simulink model "eVTOL_Small_nonandlin_algorithm_validation"  (R2024b)
settings: Solver=ode3  StartTime=0.0  StopTime=220  FixedStep=0.02  RelTol=1e-3
undefined symbols (not defined in the file): a_, b, c, c1_, deg, dttrim0, F, g, g1, h1, l1, m, MIL, PARAR, rad, rho, s, T, u_dim, ut, x_dim, xf, xmset, y_dim, yf, ymset, zf, zmset
libraries: simulink x34, aerolibconvert2 x5, aerolibwind2 x2, shared6dof x1
(part 6 of 7)

== matlab function eVTOL_Small_nonandlin_algorithm_validation/各部件气动力和力矩/8组旋翼模块/旋翼组7/上旋翼7  ==
  data: FMx output; omegaset input; u input; v input; w input; p input; q input; r input; xmset input; ymset input; zmset input; PARAR input; FMy output; FMz output; MMx output; MMy output; MMz output; PSR output; viU output; AEOCTB output
 function [FMx, FMy, FMz, MMx, MMy, MMz, PSR, viU, AEOCTB] = ROTOR7U(omegaset,u,v,w,p,q,r,xmset,ymset,zmset,PARAR) 

 % omegaset(7)为第七组上旋翼
 omega = omegaset(7);
  
 % 需要的无量纲和旋翼参数
 kt = 0.01;
 
 d2r = 0.017453292;
 
 rho = PARAR(1);
 eta = PARAR(2);
 g   = PARAR(3);
 
 nbMR     =  PARAR(4);                   % 桨叶片数(Number of blades)
 RM       =  PARAR(5);                   % 桨叶半径(Rotor radius), m
 cMR      =  PARAR(6);                   % 桨叶弦长(Blade root chord), m
 eMR      =  PARAR(7);                   % 挥舞铰偏置量(Flapping hinge offset), m
 isMR     =  PARAR(8);                   % 旋翼前倾角(Rotor shaft tilt), rad
 MbMR     =  PARAR(9);                   % 单片桨叶关于挥舞铰的质量矩(Mass moment of blade about flapping hinge), kg*m
 IbMR     =  PARAR(10);                  % 单片桨叶关于挥舞铰的惯性矩(Inertia moment of blade about flapping hinge), kg*m^2
 KindMRU  =  PARAR(11);                  % 上旋翼诱导功率修正系数;
 interU   =  PARAR(12);                  % 上旋翼诱导速度修正系数;
 interL   =  PARAR(13);                  % 下旋翼诱导速度修正系数;
 KindMR   =  PARAR(14);                  % 诱导功率修正系数(Induced power factor)
 XKBR     =  PARAR(15);                  % 桨叶挥舞弹簧系数(N-M/RAD)
 theta1MR =  PARAR(16);                  % 桨叶扭转角(Blade twist), rad
 aMR      =  PARAR(17);                  % 桨叶升力线斜率(Blade lift curve slope)
 cdMR     =  PARAR(18);                  % 单片桨叶的型阻系数(Blade profile drag coefficient)
 kBLADE   =  PARAR(19);                  % 叶端损失系数
 sigmaMR  =  PARAR(20);                  % 旋翼实度(Rotor solidity)
 gamaMR   =  PARAR(21);                  % 桨叶洛克数(Blade Lock number)

 xm = xmset(7); % 旋翼桨毂中心位置，第七组旋翼
 ym = ymset(7);
 zm = zmset(7);
 
 theta0 = PARAR(22);
 thetac = PARAR(23);
 thetas = PARAR(24);
 
 % 1.体轴系重心速度 转换到 体轴系桨毂处的速度
 uM  = u + (zm*q - ym*r);
 vM  = v + (xm*r - zm*p);
 wM  = w + (ym*p - xm*q);
 
 % 2.体轴系桨毂处的速度 转换到 桨毂轴系速度（无量纲）  直升机运动速度，不是风的速度
 muxB = ( uM*cos(isMR) + wM*sin(isMR) )/(omega*RM);   % m/s /(omega*RM)
 muyB = ( vM )/(omega*RM);                            % m/s /(omega*RM)
 muzB = (-uM*sin(isMR) + wM*cos(isMR) )/(omega*RM);   % m/s /(omega*RM)
 
 % 3.体轴系桨毂处的角速度 转换到 桨毂轴系角速度（无量纲） 确定旋翼锥度角、后倒角和侧倾角,还有后向力系数与侧向力系数
 wxB  = ( p*cos(isMR) + r*sin(isMR) )/omega;    % rad/s /(omega)
 wyB  = ( q )/omega;
 %wzB  = (-p*sin(isMR) + r*cos(isMR) )/omega;
 
 % 4.初始化：确定UcB(垂直向下)，UtB(平行)
 CTB1 = 1; % CTB牛顿迭代初始值
 
 UcB  = -muzB / ( sqrt(kt*CTB1/2.d0) ); % sqrt(CT/2)*omega*R为悬停时候的诱导速度，UcB为风的速度，方向和桨毂运动速度相反，所以加上负号，搞不清楚可以假设前上飞，此时UcB一定大于0
 UtB  = sqrt(muxB^2 + muyB^2) / ( sqrt(kt*CTB1/2.d0) ); % 照道理也要添加负号，不过后面用的是Ut的平方，所以加不加负号无所谓
 
 % 5.初始化：确定诱导速度比
 if( (2.d0*UcB+3.d0)^2 + UtB*UtB >1.d0 )         % 滑流理论适用，Newton－Raphson方法迭代求解，Johson提出的涡环状态下经验估计
     viB = N_R ( UcB, UtB );                     % N_R为迭代函数
 else
     viB = UcB * ( 0.373d0*UcB*UcB + 0.598d0*UtB*UtB - 1.991d0 );
 end
 viB = viB*interU;                               % 上旋翼诱导速度修正
 
 % 6.初始化：确定fG、lammda1(无量纲)、诱导速度和AEOCTB（代数方程右端项）
 %lammda = ( UcB+viB ) * sqrt(kt*CTB1/2.d0);                % 入流速度 /(omega*RM)
 %zh      = hB*k3*RM + HR - drotor;
 mu     = sqrt(muxB^2+muyB^2);                             % /(omega*RM)
 fG     = 1.0d0; %- sigmaMR*aMR*lammda/(4.d0*kt*CTB1) * (RM/(4.d0*z))**2/( 1.d0 + (mu/lammda)**2 )
 lammda1= muzB - viB * sqrt(kt*CTB1/2.d0) * fG * KindMRU;  % 向下为正，若直升机向上飞 则muzB为负
  
 AEOCTB1  = kt*CTB1 - 0.5d0*kBLADE*aMR*sigmaMR*((1.d0/3.d0 + 0.5d0*mu^2)*theta0...
     + 0.25d0*(1.0d0 + mu^2)*theta1MR + 0.5d0*lammda1...
     - 0.5d0*(muyB*thetac + muxB*thetas) + 0.25d0*(muxB*wxB + muyB*wyB));  %  (与beta0, betac, betas无关，只与theta0, thetac, thetas有关)
 
 % 7.初始化：CTB2 = CTB1 + deltaCTB
 CTB2 = CTB1 + 1e-4;
 
 % 8.进入牛顿迭代：计算配平时候的CTB和vi
 for k = 1:10
     % 计算CTB2下的vi  
     UcB  = -muzB / ( sqrt(kt*CTB2/2.d0) );
     UtB  = sqrt(muxB^2 + muyB^2) / ( sqrt(kt*CTB2/2.d0) );
     if( (2.d0*UcB+3.d0)^2 + UtB*UtB >1.d0 )         
         viB = N_R ( UcB, UtB );                     
     else
         viB = UcB * ( 0.373d0*UcB*UcB + 0.598d0*UtB*UtB - 1.991d0 );
     end
     viB = viB*interU;
     
     % 计算CTB2下的fG、lammda1(无量纲)、诱导速度和AEOCTB（代数方程右端项）
     %lammda = ( UcB+viB ) * sqrt(kt*CTB2/2.d0);            % 入流速度 /(omega*RM)
     %zh      = hB*k3*RM + HR - drotor;
     fG     = 1.d0 ;%- sigmaMR*aMR*lammda/(4.d0*kt*CTB1) * (RM/(4.d0*z))**2/( 1.d0 + (mu/lammda)**2 )
     lammda1= muzB - viB * sqrt(kt*CTB2/2.d0) * fG * KindMRU;  % 向下为正，若直升机向上飞 则muzB为负
     
     AEOCTB2  = kt*CTB2 - 0.5d0*kBLADE*aMR*sigmaMR*((1.d0/3.d0 + 0.5d0*mu^2)*theta0...
         + 0.25d0*(1.0d0 + mu^2)*theta1MR + 0.5d0*lammda1...
         - 0.5d0*(muyB*thetac + muxB*thetas) + 0.25d0*(muxB*wxB + muyB*wyB));  %  (与beta0, betac, betas无关，只与theta0, thetac, thetas有关)
     
     dAEOCTB  =   (AEOCTB2 - AEOCTB1)/(CTB2-CTB1);
     
     AEOCTB1 = AEOCTB2;
     CTB1 = CTB2;
     CTBN = CTB2 - AEOCTB2/dAEOCTB;
     err = abs(CTBN-CTB2);
     relerr = 2*err/(abs(CTBN)+1e-4);
     CTB2 = CTBN;
     
%      % 新CTB2下的vi与AEOCTB（即y）
%      UcB  = -muzB / ( sqrt(kt*CTB2/2.d0) ); % sqrt(CT/2)*omega*R为悬停时候的诱导速度，UcB为风的速度，方向和桨毂运动速度相反，所以加上负号，搞不清楚可以假设前上飞，此时UcB一定大于0
%      UtB  = sqrt(muxB^2 + muyB^2) / ( sqrt(kt*CTB2/2.d0) ); % 照道理也要添加负号，不过后面用的是Ut的平方，所以加不加负号无所谓
%      if( (2.d0*UcB+3.d0)^2 + UtB*UtB >1.d0 )          % 滑流理论适用，Newton－Raphson方法迭代求解，Johson提出的涡环状态下经验估计
%          viB = N_R ( UcB, UtB );                      % N_R为迭代函数
%      else
%          viB = UcB * ( 0.373d0*UcB*UcB + 0.598d0*UtB*UtB - 1.991d0 );
%      end
%      viB = viB*interU;                               % 上旋翼诱导速度修正
%      %lammda = ( UcB+viB ) * sqrt(kt*CTB2/2.d0);     % 入流速度 /(omega*RM)
%      %zh      = hB*k3*RM + HR - drotor;
%      fG     = 1.d0 ;%- sigmaMR*aMR*lammda/(4.d0*kt*CTB1) * (RM/(4.d0*z))**2/( 1.d0 + (mu/lammda)**2 )
%      lammda1= muzB - viB * sqrt(kt*CTB2/2.d0) * fG * KindMR;                      % 向下为正，若直升机向上飞 则muzB为负
%      y = kt*CTB2 - 0.5d0*kBLADE*aMR*sigmaMR*((1.d0/3.d0 + 0.5d0*mu^2)*theta0...
%          + 0.25d0*(1.0d0 + mu^2)*theta1MR + 0.5d0*lammda1...
%          - 0.5d0*(muyB*thetac + muxB*thetas) + 0.25d0*(muxB*wxB + muyB*wyB));
     %if (err<1e-5)||(relerr<1e-5)||(abs(y)<1e-6)
     if (err<1e-4)||(relerr<1e-4)
         break;
     end
 end
 
 CTB = CTB2;
 vim = viB * sqrt(kt*CTB/2.d0) * fG * KindMRU;
 vim = vim*interL;                                 
 viU = vim*omega*RM;                                % 上旋翼诱导速度在下旋翼的发展
 
 AEOCTB = AEOCTB2;
 
 % 9.确定旋翼锥度角、后倒角和侧倾角(用于确定旋翼的后向力和侧向力) 
 Ca1     = 1.d0 - 0.5d0 * mu^2;
 Cb1     = 1.d0 + 0.5d0 * mu^2;
 
 beta0   = 0.5d0*kBLADE*gamaMR * ( 0.25d0*(1+mu^2)*theta0 + (0.2d0+ 1.d0/6.d0 *mu^2)*theta1MR ...
            - 1.d0/3.d0 *muyB*thetac - 1.d0/3.d0 *muxB*thetas + 1.d0/3.d0*lammda1 ...
            + 1.d0/6.d0 *muxB*wxB + 1.d0/6.d0 *muyB*wyB ) - g*MbMR/(IbMR * (omega)^2);
 
 betac   = (8.d0/3.d0 *theta0 + 2.d0*theta1MR + 2.d0*lammda1)*muxB/Ca1 ...
            - 2.d0*muxB*muyB/Ca1 *thetac - (Ca1+2.d0*muxB*muxB)/Ca1 *thetas ...
            + 4.0/(3.d0*Cb1) *muyB*beta0 ...
            + (Cb1 - muyB^2 + 16.d0/(gamaMR*kBLADE)*muxB*muyB) *wxB/(Ca1*Cb1) ...
            + (muxB*muyB - 16.d0/(gamaMR*kBLADE)*(Cb1 - muyB^2)) *wyB/(Ca1*Cb1);
 
 betas   = -(8.d0/3.d0 *theta0 + 2.d0*theta1MR + 2.d0*lammda1)*muyB/Ca1 ...
             + 2.d0*muxB*muyB/Ca1 *thetas + (Ca1+2.d0*muyB*muyB)/Ca1 *thetac ...
             + 4.0/(3.d0*Cb1) *muxB*beta0 ...
            - (Ca1 + muyB^2 - 16.d0/(gamaMR*kBLADE)*muxB*muyB) *wyB/(Ca1*Cb1) ...
            - (muxB*muyB + 16.d0/(gamaMR*kBLADE)*(Ca1 + muyB^2)) *wxB/(Ca1*Cb1);
 
 % 10.确定后向力系数、侧向力系数、需用功率
 CT = CTB*kt;
 
 CH      = 0.25d0*cdMR*sigmaMR*muxB...   % (与beta0, betac, betas, theta0, thetac, thetas均有关)
            + 0.5d0*kBLADE*aMR*sigmaMR*( ...
            (-0.75d0*muyB *beta0 + (1.0/3.d0 + 0.5d0*muyB^2) *betac + 0.5d0*muxB*muyB *betas -0.5d0*muxB*lammda1 -1.d0/6.d0*wxB) *theta0 ...
            + 0.25d0*(-2.d0*muyB *beta0 + (1.d0+muyB^2) *betac + muxB*muyB *betas -muxB*lammda1 - 0.5d0*wxB) *theta1MR ...
            + 0.5d0*((1.d0/3.d0 + muyB^2)*beta0 - muyB*betac + 0.125d0*(muyB*wxB+muxB*wyB)) *thetac ...
            + 0.25d0*(2.d0*muxB*muyB*beta0 - muxB*betac - muyB*betas + lammda1 + 0.75d0*muxB*wxB + 0.25d0*muyB*wyB) *thetas ...
            - muxB*muyB*beta0*betac - (1.d0/6.d0-muyB*muyB)*beta0*betas - 0.25d0*muyB*betac*betas + 0.25d0*muxB*(beta0^2+betac^2) ...
            + 0.75d0*(betac-2.d0*muyB*beta0)*lammda1 ...
            - 0.5d0*(lammda1+0.125d0*muxB*betac-0.875d0*muyB*betas) *wxB - 0.5d0*(1.d0/3.d0*beta0-0.625d0*muyB*betac+0.125d0*muxB*betas) *wyB );
 
 CS      = -0.25d0*cdMR*sigmaMR*muyB ... % (与beta0, betac, betas, theta0, thetac, thetas均有关)
            + 0.5d0*kBLADE*aMR*sigmaMR*( ...
            (-0.75d0*muxB *beta0 + (1.0/3.d0 + 0.5d0*muxB^2) *betas + 0.5d0*muxB*muyB *betac +0.5d0*muyB*lammda1 +1.d0/6.d0*wyB) *theta0 ...
            + 0.25d0*(-2.d0*muxB *beta0 + (1.d0+muxB^2) *betas + muxB*muyB *betac +muyB*lammda1 + 0.5d0*wyB) *theta1MR ...
            + 0.25d0*(2.d0*muxB*muyB *beta0 - muyB *betas - muxB *betac - lammda1 - 0.25d0*muxB*wxB - 0.75d0*muyB*wyB) *thetac ...
            + 0.5d0*((1.0/3.0 + muxB^2) *beta0 - muxB*betas -0.125d0*(muyB*wxB+muxB*wyB)) *thetas ...
            + muxB*muyB*beta0*betas + (1.d0/6.d0-muxB*muxB)*beta0*betac + 0.25d0*muxB*betac*betas - 0.25d0*muyB*(beta0^2+betas^2) ...
            + 0.75d0*(betas-2.d0*muxB*beta0)*lammda1 ...
            + 0.5d0*(lammda1-0.125d0*muyB*betas+0.875d0*muxB*betac) *wyB - 0.5d0*(1.d0/3.d0*beta0-0.625d0*muxB*betas+0.125d0*muyB*betac) *wxB );
 
 CHB      =  CH / kt;
 CSB      =  CS / kt;
 
 CpmB = (-CTB*muzB - CHB*muxB + CSB*muyB)/sqrt(kt) + KindMRU*fG*CTB*sqrt(CTB/2.d0)*viB/interU ...
         + 0.125d0*sigmaMR*cdMR/kt/sqrt(kt)*(1.d0 + 4.7d0*mu^2);

 Cpm = CpmB*(kt*sqrt(kt));
      
 PSR = 1/eta*rho*(pi*RM^2)*(omega*RM)^3*Cpm;
 
 MMk = PSR/omega;
 
 TLHK = nbMR/2.d0 * (XKBR)*betas;
 TMHK = nbMR/2.d0 * (XKBR)*betac;
 
 % 11.确定体轴系下的力和力矩
 FMx =  rho*(pi*RM^2)*(omega*RM)^2 * ( CT*sin(isMR) - CH*cos(isMR) );
 
 FMy =  rho*(pi*RM^2)*(omega*RM)^2 * CS;
 
 FMz = -rho*(pi*RM^2)*(omega*RM)^2 * ( CT*cos(isMR) + CH*sin(isMR) );
 
 MMx = 0.5*nbMR * MbMR * omega^2 * eMR * betas*cos(isMR) - MMk*sin(isMR)  + ( ym*FMz - zm*FMy ) + TLHK*cos(isMR);
 
 MMy = 0.5*nbMR * MbMR * omega^2 * eMR * betac + ( zm*FMx - xm*FMz ) + TMHK;
 
 MMz = 0.5*nbMR * MbMR * omega^2 * eMR * betas*sin(isMR) + MMk*cos(isMR)  + ( xm*FMy - ym*FMx ) + TLHK*sin(isMR);

 
 % 求诱导速度用到的函数
     function p0 = N_R(x_1B,x_2B)
         p0   = 1;
         delta= 0.0001;
         epsilon = 0.0001;
         max1 = 10;
         for k = 1:max1
             p1     = p0-( p0^4+2*x_1B*p0^3+(x_1B^2+x_2B^2)*p0^2-1 )/( 4*p0^3+6*x_1B*p0^2+2*(x_1B^2+x_2B^2)*p0 );
             err    = abs(p1-p0);
             relerr = 2*err/(abs(p1)+delta);
             p0     = p1;
             y      = p0^4+2*x_1B*p0^3+(x_1B^2+x_2B^2)*p0^2-1;
             if (err<delta)||(relerr<delta)||(abs(y)<epsilon)
                 break;
             end
         end

== matlab function eVTOL_Small_nonandlin_algorithm_validation/Voltage_drop ==
  data: Vcoff output; Vcurrent input; dttrim output
function  [Vcoff,dttrim] = voltage_drop(Vcurrent)

Vcurrent1 = Vcurrent + 4;

% 本代码用于压降拟合；
% 根据二代机压降的数据整理可知，相同油门下，转速随电压基本呈现线性变化（详见一二代机压降关系表）；
% 根据零代机的实际试飞情况，满电状态（61V），悬停所需motormax=1.005；低电状态（52V），悬停所需motormax接近1.28（92%油门）；
% 满电状态下的motor与上下旋翼转速之间的关系已经通过旋翼台测得；
% 低电状态下的dt已知，根据线性变化假设，此时悬停对应的转速可以通过满电时候的转速乘以一个系数Vcoff获得（让motormax=1.28时悬停）；
% 最终可以获得低电状态下motor与上下旋翼转速之间的关系，利用不同电压下转速的线性插值，即可反推悬停时候的dt，即不同电压下的dt配平值；

dttrim = 0.0010778*Vcurrent1^2 - 0.14794*Vcurrent1 + 5.888;

Vcoff = 1; %0.011343*Vcurrent1 + 0.30803;

== matlab function eVTOL_Small_nonandlin_algorithm_validation/各部件气动力和力矩/8组旋翼模块/旋翼组7/下旋翼7 ==
  data: FMx output; omegaset input; u input; v input; w input; p input; q input; r input; xmset input; ymset input; zmset input; FMy output; FMz output; MMx output; MMy output; MMz output; PSR output; viL output; AEOCTB output; PARAR input; viU input
 function [FMx, FMy, FMz, MMx, MMy, MMz, PSR, viL, AEOCTB] = ROTOR7L(omegaset,u,v,w,p,q,r,xmset,ymset,zmset,PARAR,viU) 

 % omegaset(15)为第七组下旋翼
 omega = omegaset(15);
  
 % 需要的无量纲和旋翼参数
 kt = 0.01;
 
 d2r = 0.017453292;
 
 rho = PARAR(1);
 eta = PARAR(2);
 g   = PARAR(3);
 
 nbMR     =  PARAR(4);                   % 桨叶片数(Number of blades)
 RM       =  PARAR(5);                   % 桨叶半径(Rotor radius), m
 cMR      =  PARAR(6);                   % 桨叶弦长(Blade root chord), m
 eMR      =  PARAR(7);                   % 挥舞铰偏置量(Flapping hinge offset), m
 isMR     =  PARAR(8);                   % 旋翼前倾角(Rotor shaft tilt), rad
 MbMR     =  PARAR(9);                   % 单片桨叶关于挥舞铰的质量矩(Mass moment of blade about flapping hinge), kg*m
 IbMR     =  PARAR(10);                  % 单片桨叶关于挥舞铰的惯性矩(Inertia moment of blade about flapping hinge), kg*m^2
 KindMR   =  PARAR(14);                  % 诱导功率修正系数(Induced power factor)
 XKBR     =  PARAR(15);                  % 桨叶挥舞弹簧系数(N-M/RAD)
 theta1MR =  PARAR(16);                  % 桨叶扭转角(Blade twist), rad
 aMR      =  PARAR(17);                  % 桨叶升力线斜率(Blade lift curve slope)
 cdMR     =  PARAR(18);                  % 单片桨叶的型阻系数(Blade profile drag coefficient)
 kBLADE   =  PARAR(19);                  % 叶端损失系数
 sigmaMR  =  PARAR(20);                  % 旋翼实度(Rotor solidity)
 gamaMR   =  PARAR(21);                  % 桨叶洛克数(Blade Lock number)
 drotor   =  PARAR(25);                  % 上下旋翼间距, m
 cdMRL    =  PARAR(26);                  % 下旋翼单片桨叶的型阻系数(Blade profile drag coefficient)

 xm = xmset(7); % 旋翼桨毂中心位置，第七组旋翼
 ym = ymset(7);
 zm = zmset(7);
 
 zm = zm + drotor;
 
 theta0 = PARAR(22);
 thetac = PARAR(23);
 thetas = PARAR(24);
 
 % 1.体轴系重心速度 转换到 体轴系桨毂处的速度（无量纲）
 uM  = u + (zm*q - ym*r);
 vM  = v + (xm*r - zm*p);
 wM  = w + (ym*p - xm*q);
 
 % 2.体轴系桨毂处的速度 转换到 桨毂轴系速度（无量纲）  直升机运动速度，不是风的速度
 muxB = ( uM*cos(isMR) + wM*sin(isMR) )/(omega*RM);                     % m/s /(omega*RM)
 muyB = ( vM )/(omega*RM);                                              % m/s /(omega*RM)
 muzB = (-uM*sin(isMR) + wM*cos(isMR) )/(omega*RM) - viU/(omega*RM);    % m/s /(omega*RM)
 
 %muyB = -muyB; % 左旋翼（顺时针）中的muyB作用与右旋翼（逆时针）相反
 
 % 3.体轴系桨毂处的角速度 转换到 桨毂轴系角速度（无量纲） 确定旋翼锥度角、后倒角和侧倾角,还有后向力系数与侧向力系数
 wxB  = ( p*cos(isMR) + r*sin(isMR) )/(omega);    % rad/s /(omega)
 wyB  = ( q )/(omega);
 %wzB  = (-pB*sin(isMR) + rB*cos(isMR) )/(omega);
 
 %wxB  = -wxB; % 左旋翼（顺时针）中的wxB作用与右旋翼（逆时针）相反
 %wzB  = -wzB; % 转换为左旋翼坐标，wzB的方向相反
 
 % 4.初始化：确定UcB(垂直向下)，UtB(平行)
 CTB1 = 1; % CTB牛顿迭代初始值
 
 UcB  = -muzB / ( sqrt(kt*CTB1/2.d0) ); % sqrt(CT/2)*omega*R为悬停时候的诱导速度，UcB为风的速度，方向和桨毂运动速度相反，所以加上负号，搞不清楚可以假设前上飞，此时UcB一定大于0
 UtB  = sqrt(muxB^2 + muyB^2) / ( sqrt(kt*CTB1/2.d0) ); % 照道理也要添加负号，不过后面用的是Ut的平方，所以加不加负号无所谓
 
 % 5.初始化：确定诱导速度比
 if( (2.d0*UcB+3.d0)^2 + UtB*UtB >1.d0 )         % 滑流理论适用，Newton－Raphson方法迭代求解，Johson提出的涡环状态下经验估计
     viB = N_R ( UcB, UtB );                     % N_R为迭代函数
 else
     viB = UcB * ( 0.373d0*UcB*UcB + 0.598d0*UtB*UtB - 1.991d0 );
 end
 
 % 6.初始化：确定fG、lammda1(无量纲)、诱导速度和AEOCTB（代数方程右端项）
 %lammda = ( UcB+viB ) * sqrt(kt*CTB1/2.d0);                % 入流速度 /(omega*RM)
 %zh      = hB*k3*RM + HR - drotor;
 mu     = sqrt(muxB^2+muyB^2);                             % /(omega*RM)
 fG     = 1.0d0; %- sigmaMR*aMR*lammda/(4.d0*kt*CTB1) * (RM/(4.d0*z))**2/( 1.d0 + (mu/lammda)**2 )
 lammda1= muzB - viB * sqrt(kt*CTB1/2.d0) * fG * KindMR;  % 向下为正，若直升机向上飞 则muzB为负
  
 AEOCTB1  = kt*CTB1 - 0.5d0*kBLADE*aMR*sigmaMR*((1.d0/3.d0 + 0.5d0*mu^2)*theta0...
     + 0.25d0*(1.0d0 + mu^2)*theta1MR + 0.5d0*lammda1...
     - 0.5d0*(muyB*thetac + muxB*thetas) + 0.25d0*(muxB*wxB + muyB*wyB));  %  (与beta0, betac, betas无关，只与theta0, thetac, thetas有关)
 
 % 7.初始化：CTB2 = CTB1 + deltaCTB
 CTB2 = CTB1 + 1e-4;
 
 % 8.进入牛顿迭代：计算配平时候的CTB和vi
 for k = 1:10
     % 计算CTB2下的vi  
     UcB  = -muzB / ( sqrt(kt*CTB2/2.d0) );
     UtB  = sqrt(muxB^2 + muyB^2) / ( sqrt(kt*CTB2/2.d0) );
     if( (2.d0*UcB+3.d0)^2 + UtB*UtB >1.d0 )         
         viB = N_R ( UcB, UtB );                     
     else
         viB = UcB * ( 0.373d0*UcB*UcB + 0.598d0*UtB*UtB - 1.991d0 );
     end
     
     % 计算CTB2下的fG、lammda1(无量纲)、诱导速度和AEOCTB（代数方程右端项）
     %lammda = ( UcB+viB ) * sqrt(kt*CTB2/2.d0);            % 入流速度 /(omega*RM)
     %zh      = hB*k3*RM + HR - drotor;
     fG     = 1.d0 ;%- sigmaMR*aMR*lammda/(4.d0*kt*CTB1) * (RM/(4.d0*z))**2/( 1.d0 + (mu/lammda)**2 )
     lammda1= muzB - viB * sqrt(kt*CTB2/2.d0) * fG * KindMR;  % 向下为正，若直升机向上飞 则muzB为负
     
     AEOCTB2  = kt*CTB2 - 0.5d0*kBLADE*aMR*sigmaMR*((1.d0/3.d0 + 0.5d0*mu^2)*theta0...
         + 0.25d0*(1.0d0 + mu^2)*theta1MR + 0.5d0*lammda1...
         - 0.5d0*(muyB*thetac + muxB*thetas) + 0.25d0*(muxB*wxB + muyB*wyB));  %  (与beta0, betac, betas无关，只与theta0, thetac, thetas有关)
     
     dAEOCTB  =   (AEOCTB2 - AEOCTB1)/(CTB2-CTB1);
     
     AEOCTB1 = AEOCTB2;
     CTB1 = CTB2;
     CTBN = CTB2 - AEOCTB2/dAEOCTB;
     err = abs(CTBN-CTB2);
     relerr = 2*err/(abs(CTBN)+1e-4);
     CTB2 = CTBN;
     
%      % 新CTB2下的vi与AEOCTB（即y）
%      UcB  = -muzB / ( sqrt(kt*CTB2/2.d0) ); % sqrt(CT/2)*omega*R为悬停时候的诱导速度，UcB为风的速度，方向和桨毂运动速度相反，所以加上负号，搞不清楚可以假设前上飞，此时UcB一定大于0
%      UtB  = sqrt(muxB^2 + muyB^2) / ( sqrt(kt*CTB2/2.d0) ); % 照道理也要添加负号，不过后面用的是Ut的平方，所以加不加负号无所谓
%      if( (2.d0*UcB+3.d0)^2 + UtB*UtB >1.d0 )          % 滑流理论适用，Newton－Raphson方法迭代求解，Johson提出的涡环状态下经验估计
%          viB = N_R ( UcB, UtB );                      % N_R为迭代函数
%      else
%          viB = UcB * ( 0.373d0*UcB*UcB + 0.598d0*UtB*UtB - 1.991d0 );
%      end
%      %lammda = ( UcB+viB ) * sqrt(kt*CTB2/2.d0);     % 入流速度 /(omega*RM)
%      %zh      = hB*k3*RM + HR - drotor;
%      fG     = 1.d0 ;%- sigmaMR*aMR*lammda/(4.d0*kt*CTB1) * (RM/(4.d0*z))**2/( 1.d0 + (mu/lammda)**2 )
%      lammda1= muzB - viB * sqrt(kt*CTB2/2.d0) * fG * KindMR;                      % 向下为正，若直升机向上飞 则muzB为负
%      y = kt*CTB2 - 0.5d0*kBLADE*aMR*sigmaMR*((1.d0/3.d0 + 0.5d0*mu^2)*theta0...
%          + 0.25d0*(1.0d0 + mu^2)*theta1MR + 0.5d0*lammda1...
%          - 0.5d0*(muyB*thetac + muxB*thetas) + 0.25d0*(muxB*wxB + muyB*wyB));
     %if (err<1e-5)||(relerr<1e-5)||(abs(y)<1e-6)
     if (err<1e-4)||(relerr<1e-4)
         break;
     end
 end
 
 CTB = CTB2;
 vim = viB * sqrt(kt*CTB/2.d0) * fG * KindMR;
 viL = vim*omega*RM;
 
 AEOCTB = AEOCTB2;
 
 % 9.确定旋翼锥度角、后倒角和侧倾角(用于确定旋翼的后向力和侧向力) 
 Ca1     = 1.d0 - 0.5d0 * mu^2;
 Cb1     = 1.d0 + 0.5d0 * mu^2;
 
 beta0   = 0.5d0*kBLADE*gamaMR * ( 0.25d0*(1+mu^2)*theta0 + (0.2d0+ 1.d0/6.d0 *mu^2)*theta1MR ...
            - 1.d0/3.d0 *muyB*thetac - 1.d0/3.d0 *muxB*thetas + 1.d0/3.d0*lammda1 ...
            + 1.d0/6.d0 *muxB*wxB + 1.d0/6.d0 *muyB*wyB ) - g*MbMR/(IbMR * (omega)^2);
 
 betac   = (8.d0/3.d0 *theta0 + 2.d0*theta1MR + 2.d0*lammda1)*muxB/Ca1 ...
            - 2.d0*muxB*muyB/Ca1 *thetac - (Ca1+2.d0*muxB*muxB)/Ca1 *thetas ...
            + 4.0/(3.d0*Cb1) *muyB*beta0 ...
            + (Cb1 - muyB^2 + 16.d0/(gamaMR*kBLADE)*muxB*muyB) *wxB/(Ca1*Cb1) ...
            + (muxB*muyB - 16.d0/(gamaMR*kBLADE)*(Cb1 - muyB^2)) *wyB/(Ca1*Cb1);
 
 betas   = -(8.d0/3.d0 *theta0 + 2.d0*theta1MR + 2.d0*lammda1)*muyB/Ca1 ...
             + 2.d0*muxB*muyB/Ca1 *thetas + (Ca1+2.d0*muyB*muyB)/Ca1 *thetac ...
             + 4.0/(3.d0*Cb1) *muxB*beta0 ...
            - (Ca1 + muyB^2 - 16.d0/(gamaMR*kBLADE)*muxB*muyB) *wyB/(Ca1*Cb1) ...
            - (muxB*muyB + 16.d0/(gamaMR*kBLADE)*(Ca1 + muyB^2)) *wxB/(Ca1*Cb1);
 
 % 10.确定后向力系数、侧向力系数、需用功率
 CT = CTB*kt;
 
 CH      = 0.25d0*cdMRL*sigmaMR*muxB...   % (与beta0, betac, betas, theta0, thetac, thetas均有关)
            + 0.5d0*kBLADE*aMR*sigmaMR*( ...
            (-0.75d0*muyB *beta0 + (1.0/3.d0 + 0.5d0*muyB^2) *betac + 0.5d0*muxB*muyB *betas -0.5d0*muxB*lammda1 -1.d0/6.d0*wxB) *theta0 ...
            + 0.25d0*(-2.d0*muyB *beta0 + (1.d0+muyB^2) *betac + muxB*muyB *betas -muxB*lammda1 - 0.5d0*wxB) *theta1MR ...
            + 0.5d0*((1.d0/3.d0 + muyB^2)*beta0 - muyB*betac + 0.125d0*(muyB*wxB+muxB*wyB)) *thetac ...
            + 0.25d0*(2.d0*muxB*muyB*beta0 - muxB*betac - muyB*betas + lammda1 + 0.75d0*muxB*wxB + 0.25d0*muyB*wyB) *thetas ...
            - muxB*muyB*beta0*betac - (1.d0/6.d0-muyB*muyB)*beta0*betas - 0.25d0*muyB*betac*betas + 0.25d0*muxB*(beta0^2+betac^2) ...
            + 0.75d0*(betac-2.d0*muyB*beta0)*lammda1 ...
            - 0.5d0*(lammda1+0.125d0*muxB*betac-0.875d0*muyB*betas) *wxB - 0.5d0*(1.d0/3.d0*beta0-0.625d0*muyB*betac+0.125d0*muxB*betas) *wyB );
 
 CS      = -0.25d0*cdMRL*sigmaMR*muyB ... % (与beta0, betac, betas, theta0, thetac, thetas均有关)
            + 0.5d0*kBLADE*aMR*sigmaMR*( ...
            (-0.75d0*muxB *beta0 + (1.0/3.d0 + 0.5d0*muxB^2) *betas + 0.5d0*muxB*muyB *betac +0.5d0*muyB*lammda1 +1.d0/6.d0*wyB) *theta0 ...
            + 0.25d0*(-2.d0*muxB *beta0 + (1.d0+muxB^2) *betas + muxB*muyB *betac +muyB*lammda1 + 0.5d0*wyB) *theta1MR ...
            + 0.25d0*(2.d0*muxB*muyB *beta0 - muyB *betas - muxB *betac - lammda1 - 0.25d0*muxB*wxB - 0.75d0*muyB*wyB) *thetac ...
            + 0.5d0*((1.0/3.0 + muxB^2) *beta0 - muxB*betas -0.125d0*(muyB*wxB+muxB*wyB)) *thetas ...
            + muxB*muyB*beta0*betas + (1.d0/6.d0-muxB*muxB)*beta0*betac + 0.25d0*muxB*betac*betas - 0.25d0*muyB*(beta0^2+betas^2) ...
            + 0.75d0*(betas-2.d0*muxB*beta0)*lammda1 ...
            + 0.5d0*(lammda1-0.125d0*muyB*betas+0.875d0*muxB*betac) *wyB - 0.5d0*(1.d0/3.d0*beta0-0.625d0*muxB*betas+0.125d0*muyB*betac) *wxB );
 
 CHB      =  CH / kt;
 CSB      =  CS / kt;
  
 CpmB = (-CTB*muzB - CHB*muxB + CSB*muyB)/sqrt(kt) + KindMR*fG*CTB*sqrt(CTB/2.d0)*viB ...
         + 0.125d0*sigmaMR*cdMRL/kt/sqrt(kt)*(1.d0 + 4.7d0*mu^2);

 Cpm = CpmB*(kt*sqrt(kt));
      
 PSR = 1/eta*rho*(pi*RM^2)*(omega*RM)^3*Cpm;
 
 MMk = PSR/omega;
 
 %betas = -betas ; % 转换为右旋翼坐标，侧倒角betas的方向相反
 %CS   = -CS;      % 转换为右旋翼坐标，侧向力系数CS的方向相反
  
 TLHK = nbMR/2.d0 * (XKBR)*betas;
 TMHK = nbMR/2.d0 * (XKBR)*betac;
 
 % 11.确定体轴系下的力和力矩
 FMx =  rho*(pi*RM^2)*(omega*RM)^2 * ( CT*sin(isMR) - CH*cos(isMR) );
 
 FMy =  rho*(pi*RM^2)*(omega*RM)^2 * CS;
 
 FMz = -rho*(pi*RM^2)*(omega*RM)^2 * ( CT*cos(isMR) + CH*sin(isMR) );
 
 MMx = 0.5*nbMR * MbMR * omega^2 * eMR * betas*cos(isMR) - MMk*sin(isMR)  + ( ym*FMz - zm*FMy ) + TLHK*cos(isMR);
 
 MMy = 0.5*nbMR * MbMR * omega^2 * eMR * betac + ( zm*FMx - xm*FMz ) + TMHK;
 
 MMz = 0.5*nbMR * MbMR * omega^2 * eMR * betas*sin(isMR) + MMk*cos(isMR)  + ( xm*FMy - ym*FMx ) + TLHK*sin(isMR);
 
 % 求诱导速度用到的函数
     function p0 = N_R(x_1B,x_2B)
         p0   = 1;
         delta= 0.0001;
         epsilon = 0.0001;
         max1 = 10;
         for k = 1:max1
             p1     = p0-( p0^4+2*x_1B*p0^3+(x_1B^2+x_2B^2)*p0^2-1 )/( 4*p0^3+6*x_1B*p0^2+2*(x_1B^2+x_2B^2)*p0 );
             err    = abs(p1-p0);
             relerr = 2*err/(abs(p1)+delta);
             p0     = p1;
             y      = p0^4+2*x_1B*p0^3+(x_1B^2+x_2B^2)*p0^2-1;
             if (err<delta)||(relerr<delta)||(abs(y)<epsilon)
                 break;
             end
         end

== matlab function eVTOL_Small_nonandlin_algorithm_validation/各部件气动力和力矩/8组旋翼模块/旋翼组8/上旋翼8 ==
  data: FMx output; omegaset input; u input; v input; w input; p input; q input; r input; xmset input; ymset input; zmset input; PARAR input; FMy output; FMz output; MMx output; MMy output; MMz output; PSR output; viU output; AEOCTB output
 function [FMx, FMy, FMz, MMx, MMy, MMz, PSR, viU, AEOCTB] = ROTOR8U(omegaset,u,v,w,p,q,r,xmset,ymset,zmset,PARAR) 

 % omegaset(8)为第八组上旋翼
 omega = omegaset(8);
  
 % 需要的无量纲和旋翼参数
 kt = 0.01;
 
 d2r = 0.017453292;
 
 rho = PARAR(1);
 eta = PARAR(2);
 g   = PARAR(3);
 
 nbMR     =  PARAR(4);                   % 桨叶片数(Number of blades)
 RM       =  PARAR(5);                   % 桨叶半径(Rotor radius), m
 cMR      =  PARAR(6);                   % 桨叶弦长(Blade root chord), m
 eMR      =  PARAR(7);                   % 挥舞铰偏置量(Flapping hinge offset), m
 isMR     =  PARAR(8);                   % 旋翼前倾角(Rotor shaft tilt), rad
 MbMR     =  PARAR(9);                   % 单片桨叶关于挥舞铰的质量矩(Mass moment of blade about flapping hinge), kg*m
 IbMR     =  PARAR(10);                  % 单片桨叶关于挥舞铰的惯性矩(Inertia moment of blade about flapping hinge), kg*m^2
 KindMRU  =  PARAR(11);                  % 上旋翼诱导功率修正系数;
 interU   =  PARAR(12);                  % 上旋翼诱导速度修正系数;
 interL   =  PARAR(13);                  % 下旋翼诱导速度修正系数;
 KindMR   =  PARAR(14);                  % 诱导功率修正系数(Induced power factor)
 XKBR     =  PARAR(15);                  % 桨叶挥舞弹簧系数(N-M/RAD)
 theta1MR =  PARAR(16);                  % 桨叶扭转角(Blade twist), rad
 aMR      =  PARAR(17);                  % 桨叶升力线斜率(Blade lift curve slope)
 cdMR     =  PARAR(18);                  % 单片桨叶的型阻系数(Blade profile drag coefficient)
 kBLADE   =  PARAR(19);                  % 叶端损失系数
 sigmaMR  =  PARAR(20);                  % 旋翼实度(Rotor solidity)
 gamaMR   =  PARAR(21);                  % 桨叶洛克数(Blade Lock number)

 xm = xmset(8); % 旋翼桨毂中心位置，第八组旋翼
 ym = ymset(8);
 zm = zmset(8);
 
 theta0 = PARAR(22);
 thetac = PARAR(23);
 thetas = PARAR(24);
 
 % 1.体轴系重心速度 转换到 体轴系桨毂处的速度
 uM  = u + (zm*q - ym*r);
 vM  = v + (xm*r - zm*p);
 wM  = w + (ym*p - xm*q);
 
 % 2.体轴系桨毂处的速度 转换到 桨毂轴系速度（无量纲）  直升机运动速度，不是风的速度
 muxB = ( uM*cos(isMR) + wM*sin(isMR) )/(omega*RM);   % m/s /(omega*RM)
 muyB = ( vM )/(omega*RM);                            % m/s /(omega*RM)
 muzB = (-uM*sin(isMR) + wM*cos(isMR) )/(omega*RM);   % m/s /(omega*RM)
 
 muyB = -muyB; % 左旋翼（顺时针）中的muyB作用与右旋翼（逆时针）相反
 
 % 3.体轴系桨毂处的角速度 转换到 桨毂轴系角速度（无量纲） 确定旋翼锥度角、后倒角和侧倾角,还有后向力系数与侧向力系数
 wxB  = ( p*cos(isMR) + r*sin(isMR) )/omega;    % rad/s /(omega)
 wyB  = ( q )/omega;
 %wzB  = (-p*sin(isMR) + r*cos(isMR) )/omega;
 
 wxB  = -wxB; % 左旋翼（顺时针）中的wxB作用与右旋翼（逆时针）相反
 %wzB  = -wzB; % 转换为左旋翼坐标，wzB的方向相反
 
 % 4.初始化：确定UcB(垂直向下)，UtB(平行)
 CTB1 = 1; % CTB牛顿迭代初始值
 
 UcB  = -muzB / ( sqrt(kt*CTB1/2.d0) ); % sqrt(CT/2)*omega*R为悬停时候的诱导速度，UcB为风的速度，方向和桨毂运动速度相反，所以加上负号，搞不清楚可以假设前上飞，此时UcB一定大于0
 UtB  = sqrt(muxB^2 + muyB^2) / ( sqrt(kt*CTB1/2.d0) ); % 照道理也要添加负号，不过后面用的是Ut的平方，所以加不加负号无所谓
 
 % 5.初始化：确定诱导速度比
 if( (2.d0*UcB+3.d0)^2 + UtB*UtB >1.d0 )         % 滑流理论适用，Newton－Raphson方法迭代求解，Johson提出的涡环状态下经验估计
     viB = N_R ( UcB, UtB );                     % N_R为迭代函数
 else
     viB = UcB * ( 0.373d0*UcB*UcB + 0.598d0*UtB*UtB - 1.991d0 );
 end
 viB = viB*interU;                               % 上旋翼诱导速度修正
 
 % 6.初始化：确定fG、lammda1(无量纲)、诱导速度和AEOCTB（代数方程右端项）
 %lammda = ( UcB+viB ) * sqrt(kt*CTB1/2.d0);                % 入流速度 /(omega*RM)
 %zh      = hB*k3*RM + HR - drotor;
 mu     = sqrt(muxB^2+muyB^2);                             % /(omega*RM)
 fG     = 1.0d0; %- sigmaMR*aMR*lammda/(4.d0*kt*CTB1) * (RM/(4.d0*z))**2/( 1.d0 + (mu/lammda)**2 )
 lammda1= muzB - viB * sqrt(kt*CTB1/2.d0) * fG * KindMRU;  % 向下为正，若直升机向上飞 则muzB为负
  
 AEOCTB1  = kt*CTB1 - 0.5d0*kBLADE*aMR*sigmaMR*((1.d0/3.d0 + 0.5d0*mu^2)*theta0...
     + 0.25d0*(1.0d0 + mu^2)*theta1MR + 0.5d0*lammda1...
     - 0.5d0*(muyB*thetac + muxB*thetas) + 0.25d0*(muxB*wxB + muyB*wyB));  %  (与beta0, betac, betas无关，只与theta0, thetac, thetas有关)
 
 % 7.初始化：CTB2 = CTB1 + deltaCTB
 CTB2 = CTB1 + 1e-4;
 
 % 8.进入牛顿迭代：计算配平时候的CTB和vi
 for k = 1:10
     % 计算CTB2下的vi  
     UcB  = -muzB / ( sqrt(kt*CTB2/2.d0) );
     UtB  = sqrt(muxB^2 + muyB^2) / ( sqrt(kt*CTB2/2.d0) );
     if( (2.d0*UcB+3.d0)^2 + UtB*UtB >1.d0 )         
         viB = N_R ( UcB, UtB );                     
     else
         viB = UcB * ( 0.373d0*UcB*UcB + 0.598d0*UtB*UtB - 1.991d0 );
     end
     viB = viB*interU;
     
     % 计算CTB2下的fG、lammda1(无量纲)、诱导速度和AEOCTB（代数方程右端项）
     %lammda = ( UcB+viB ) * sqrt(kt*CTB2/2.d0);            % 入流速度 /(omega*RM)
     %zh      = hB*k3*RM + HR - drotor;
     fG     = 1.d0 ;%- sigmaMR*aMR*lammda/(4.d0*kt*CTB1) * (RM/(4.d0*z))**2/( 1.d0 + (mu/lammda)**2 )
     lammda1= muzB - viB * sqrt(kt*CTB2/2.d0) * fG * KindMRU;  % 向下为正，若直升机向上飞 则muzB为负
     
     AEOCTB2  = kt*CTB2 - 0.5d0*kBLADE*aMR*sigmaMR*((1.d0/3.d0 + 0.5d0*mu^2)*theta0...
         + 0.25d0*(1.0d0 + mu^2)*theta1MR + 0.5d0*lammda1...
         - 0.5d0*(muyB*thetac + muxB*thetas) + 0.25d0*(muxB*wxB + muyB*wyB));  %  (与beta0, betac, betas无关，只与theta0, thetac, thetas有关)
     
     dAEOCTB  =   (AEOCTB2 - AEOCTB1)/(CTB2-CTB1);
     
     AEOCTB1 = AEOCTB2;
     CTB1 = CTB2;
     CTBN = CTB2 - AEOCTB2/dAEOCTB;
     err = abs(CTBN-CTB2);
     relerr = 2*err/(abs(CTBN)+1e-4);
     CTB2 = CTBN;
     
%      % 新CTB2下的vi与AEOCTB（即y）
%      UcB  = -muzB / ( sqrt(kt*CTB2/2.d0) ); % sqrt(CT/2)*omega*R为悬停时候的诱导速度，UcB为风的速度，方向和桨毂运动速度相反，所以加上负号，搞不清楚可以假设前上飞，此时UcB一定大于0
%      UtB  = sqrt(muxB^2 + muyB^2) / ( sqrt(kt*CTB2/2.d0) ); % 照道理也要添加负号，不过后面用的是Ut的平方，所以加不加负号无所谓
%      if( (2.d0*UcB+3.d0)^2 + UtB*UtB >1.d0 )          % 滑流理论适用，Newton－Raphson方法迭代求解，Johson提出的涡环状态下经验估计
%          viB = N_R ( UcB, UtB );                      % N_R为迭代函数
%      else
%          viB = UcB * ( 0.373d0*UcB*UcB + 0.598d0*UtB*UtB - 1.991d0 );
%      end
%      viB = viB*interU;                               % 上旋翼诱导速度修正
%      %lammda = ( UcB+viB ) * sqrt(kt*CTB2/2.d0);     % 入流速度 /(omega*RM)
%      %zh      = hB*k3*RM + HR - drotor;
%      fG     = 1.d0 ;%- sigmaMR*aMR*lammda/(4.d0*kt*CTB1) * (RM/(4.d0*z))**2/( 1.d0 + (mu/lammda)**2 )
%      lammda1= muzB - viB * sqrt(kt*CTB2/2.d0) * fG * KindMR;                      % 向下为正，若直升机向上飞 则muzB为负
%      y = kt*CTB2 - 0.5d0*kBLADE*aMR*sigmaMR*((1.d0/3.d0 + 0.5d0*mu^2)*theta0...
%          + 0.25d0*(1.0d0 + mu^2)*theta1MR + 0.5d0*lammda1...
%          - 0.5d0*(muyB*thetac + muxB*thetas) + 0.25d0*(muxB*wxB + muyB*wyB));
     %if (err<1e-5)||(relerr<1e-5)||(abs(y)<1e-6)
     if (err<1e-4)||(relerr<1e-4)
         break;
     end
 end
 
 CTB = CTB2;
 vim = viB * sqrt(kt*CTB/2.d0) * fG * KindMRU;
 vim = vim*interL;                                 
 viU = vim*omega*RM;                                % 上旋翼诱导速度在下旋翼的发展
 
 AEOCTB = AEOCTB2;
 
 % 9.确定旋翼锥度角、后倒角和侧倾角(用于确定旋翼的后向力和侧向力) 
 Ca1     = 1.d0 - 0.5d0 * mu^2;
 Cb1     = 1.d0 + 0.5d0 * mu^2;
 
 beta0   = 0.5d0*kBLADE*gamaMR * ( 0.25d0*(1+mu^2)*theta0 + (0.2d0+ 1.d0/6.d0 *mu^2)*theta1MR ...
            - 1.d0/3.d0 *muyB*thetac - 1.d0/3.d0 *muxB*thetas + 1.d0/3.d0*lammda1 ...
            + 1.d0/6.d0 *muxB*wxB + 1.d0/6.d0 *muyB*wyB ) - g*MbMR/(IbMR * (omega)^2);
 
 betac   = (8.d0/3.d0 *theta0 + 2.d0*theta1MR + 2.d0*lammda1)*muxB/Ca1 ...
            - 2.d0*muxB*muyB/Ca1 *thetac - (Ca1+2.d0*muxB*muxB)/Ca1 *thetas ...
            + 4.0/(3.d0*Cb1) *muyB*beta0 ...
            + (Cb1 - muyB^2 + 16.d0/(gamaMR*kBLADE)*muxB*muyB) *wxB/(Ca1*Cb1) ...
            + (muxB*muyB - 16.d0/(gamaMR*kBLADE)*(Cb1 - muyB^2)) *wyB/(Ca1*Cb1);
 
 betas   = -(8.d0/3.d0 *theta0 + 2.d0*theta1MR + 2.d0*lammda1)*muyB/Ca1 ...
             + 2.d0*muxB*muyB/Ca1 *thetas + (Ca1+2.d0*muyB*muyB)/Ca1 *thetac ...
             + 4.0/(3.d0*Cb1) *muxB*beta0 ...
            - (Ca1 + muyB^2 - 16.d0/(gamaMR*kBLADE)*muxB*muyB) *wyB/(Ca1*Cb1) ...
            - (muxB*muyB + 16.d0/(gamaMR*kBLADE)*(Ca1 + muyB^2)) *wxB/(Ca1*Cb1);
 
 % 10.确定后向力系数、侧向力系数、需用功率
 CT = CTB*kt;
 
 CH      = 0.25d0*cdMR*sigmaMR*muxB...   % (与beta0, betac, betas, theta0, thetac, thetas均有关)
            + 0.5d0*kBLADE*aMR*sigmaMR*( ...
            (-0.75d0*muyB *beta0 + (1.0/3.d0 + 0.5d0*muyB^2) *betac + 0.5d0*muxB*muyB *betas -0.5d0*muxB*lammda1 -1.d0/6.d0*wxB) *theta0 ...
            + 0.25d0*(-2.d0*muyB *beta0 + (1.d0+muyB^2) *betac + muxB*muyB *betas -muxB*lammda1 - 0.5d0*wxB) *theta1MR ...
            + 0.5d0*((1.d0/3.d0 + muyB^2)*beta0 - muyB*betac + 0.125d0*(muyB*wxB+muxB*wyB)) *thetac ...
            + 0.25d0*(2.d0*muxB*muyB*beta0 - muxB*betac - muyB*betas + lammda1 + 0.75d0*muxB*wxB + 0.25d0*muyB*wyB) *thetas ...
            - muxB*muyB*beta0*betac - (1.d0/6.d0-muyB*muyB)*beta0*betas - 0.25d0*muyB*betac*betas + 0.25d0*muxB*(beta0^2+betac^2) ...
            + 0.75d0*(betac-2.d0*muyB*beta0)*lammda1 ...
            - 0.5d0*(lammda1+0.125d0*muxB*betac-0.875d0*muyB*betas) *wxB - 0.5d0*(1.d0/3.d0*beta0-0.625d0*muyB*betac+0.125d0*muxB*betas) *wyB );
 
 CS      = -0.25d0*cdMR*sigmaMR*muyB ... % (与beta0, betac, betas, theta0, thetac, thetas均有关)
            + 0.5d0*kBLADE*aMR*sigmaMR*( ...
            (-0.75d0*muxB *beta0 + (1.0/3.d0 + 0.5d0*muxB^2) *betas + 0.5d0*muxB*muyB *betac +0.5d0*muyB*lammda1 +1.d0/6.d0*wyB) *theta0 ...
            + 0.25d0*(-2.d0*muxB *beta0 + (1.d0+muxB^2) *betas + muxB*muyB *betac +muyB*lammda1 + 0.5d0*wyB) *theta1MR ...
            + 0.25d0*(2.d0*muxB*muyB *beta0 - muyB *betas - muxB *betac - lammda1 - 0.25d0*muxB*wxB - 0.75d0*muyB*wyB) *thetac ...
            + 0.5d0*((1.0/3.0 + muxB^2) *beta0 - muxB*betas -0.125d0*(muyB*wxB+muxB*wyB)) *thetas ...
            + muxB*muyB*beta0*betas + (1.d0/6.d0-muxB*muxB)*beta0*betac + 0.25d0*muxB*betac*betas - 0.25d0*muyB*(beta0^2+betas^2) ...
            + 0.75d0*(betas-2.d0*muxB*beta0)*lammda1 ...
            + 0.5d0*(lammda1-0.125d0*muyB*betas+0.875d0*muxB*betac) *wyB - 0.5d0*(1.d0/3.d0*beta0-0.625d0*muxB*betas+0.125d0*muyB*betac) *wxB );
 
 CHB      =  CH / kt;
 CSB      =  CS / kt;
 
 CpmB = (-CTB*muzB - CHB*muxB + CSB*muyB)/sqrt(kt) + KindMRU*fG*CTB*sqrt(CTB/2.d0)*viB/interU ...
         + 0.125d0*sigmaMR*cdMR/kt/sqrt(kt)*(1.d0 + 4.7d0*mu^2);

 Cpm = CpmB*(kt*sqrt(kt));
      
 PSR = 1/eta*rho*(pi*RM^2)*(omega*RM)^3*Cpm;
 
 MMk = -PSR/omega;
 
 betas = -betas ; % 转换为右旋翼坐标，侧倒角betas的方向相反
 CS   = -CS;      % 转换为右旋翼坐标，侧向力系数CS的方向相反
 
 TLHK = nbMR/2.d0 * (XKBR)*betas;
 TMHK = nbMR/2.d0 * (XKBR)*betac;
 
 % 11.确定体轴系下的力和力矩
 FMx =  rho*(pi*RM^2)*(omega*RM)^2 * ( CT*sin(isMR) - CH*cos(isMR) );
 
 FMy =  rho*(pi*RM^2)*(omega*RM)^2 * CS;
 
 FMz = -rho*(pi*RM^2)*(omega*RM)^2 * ( CT*cos(isMR) + CH*sin(isMR) );
 
 MMx = 0.5*nbMR * MbMR * omega^2 * eMR * betas*cos(isMR) - MMk*sin(isMR)  + ( ym*FMz - zm*FMy ) + TLHK*cos(isMR);
 
 MMy = 0.5*nbMR * MbMR * omega^2 * eMR * betac + ( zm*FMx - xm*FMz ) + TMHK;
 
 MMz = 0.5*nbMR * MbMR * omega^2 * eMR * betas*sin(isMR) + MMk*cos(isMR)  + ( xm*FMy - ym*FMx ) + TLHK*sin(isMR);

 
 % 求诱导速度用到的函数
     function p0 = N_R(x_1B,x_2B)
         p0   = 1;
         delta= 0.0001;
         epsilon = 0.0001;
         max1 = 10;
         for k = 1:max1
             p1     = p0-( p0^4+2*x_1B*p0^3+(x_1B^2+x_2B^2)*p0^2-1 )/( 4*p0^3+6*x_1B*p0^2+2*(x_1B^2+x_2B^2)*p0 );
             err    = abs(p1-p0);
             relerr = 2*err/(abs(p1)+delta);
             p0     = p1;
             y      = p0^4+2*x_1B*p0^3+(x_1B^2+x_2B^2)*p0^2-1;
             if (err<delta)||(relerr<delta)||(abs(y)<epsilon)
                 break;
             end
         end

== matlab function eVTOL_Small_nonandlin_algorithm_validation/各部件气动力和力矩/8组旋翼模块/旋翼组8/下旋翼8 ==
  data: FMx output; omegaset input; u input; v input; w input; p input; q input; r input; xmset input; ymset input; zmset input; FMy output; FMz output; MMx output; MMy output; MMz output; PSR output; viL output; AEOCTB output; PARAR input; viU input
 function [FMx, FMy, FMz, MMx, MMy, MMz, PSR, viL, AEOCTB] = ROTOR8L(omegaset,u,v,w,p,q,r,xmset,ymset,zmset,PARAR,viU) 

 % omegaset(16)为第八组下旋翼
 omega = omegaset(16);
  
 % 需要的无量纲和旋翼参数
 kt = 0.01;
 
 d2r = 0.017453292;
 
 rho = PARAR(1);
 eta = PARAR(2);
 g   = PARAR(3);
 
 nbMR     =  PARAR(4);                   % 桨叶片数(Number of blades)
 RM       =  PARAR(5);                   % 桨叶半径(Rotor radius), m
 cMR      =  PARAR(6);                   % 桨叶弦长(Blade root chord), m
 eMR      =  PARAR(7);                   % 挥舞铰偏置量(Flapping hinge offset), m
 isMR     =  PARAR(8);                   % 旋翼前倾角(Rotor shaft tilt), rad
 MbMR     =  PARAR(9);                   % 单片桨叶关于挥舞铰的质量矩(Mass moment of blade about flapping hinge), kg*m
 IbMR     =  PARAR(10);                  % 单片桨叶关于挥舞铰的惯性矩(Inertia moment of blade about flapping hinge), kg*m^2
 KindMR   =  PARAR(14);                  % 诱导功率修正系数(Induced power factor)
 XKBR     =  PARAR(15);                  % 桨叶挥舞弹簧系数(N-M/RAD)
 theta1MR =  PARAR(16);                  % 桨叶扭转角(Blade twist), rad
 aMR      =  PARAR(17);                  % 桨叶升力线斜率(Blade lift curve slope)
 cdMR     =  PARAR(18);                  % 单片桨叶的型阻系数(Blade profile drag coefficient)
 kBLADE   =  PARAR(19);                  % 叶端损失系数
 sigmaMR  =  PARAR(20);                  % 旋翼实度(Rotor solidity)
 gamaMR   =  PARAR(21);                  % 桨叶洛克数(Blade Lock number)
 drotor   =  PARAR(25);                  % 上下旋翼间距, m
 cdMRL    =  PARAR(26);                  % 下旋翼单片桨叶的型阻系数(Blade profile drag coefficient)

 xm = xmset(8); % 旋翼桨毂中心位置，第八组旋翼
 ym = ymset(8);
 zm = zmset(8);
 
 zm = zm + drotor;
 
 theta0 = PARAR(22);
 thetac = PARAR(23);
 thetas = PARAR(24);
 
 % 1.体轴系重心速度 转换到 体轴系桨毂处的速度（无量纲）
 uM  = u + (zm*q - ym*r);
 vM  = v + (xm*r - zm*p);
 wM  = w + (ym*p - xm*q);
 
 % 2.体轴系桨毂处的速度 转换到 桨毂轴系速度（无量纲）  直升机运动速度，不是风的速度
 muxB = ( uM*cos(isMR) + wM*sin(isMR) )/(omega*RM);                     % m/s /(omega*RM)
 muyB = ( vM )/(omega*RM);                                              % m/s /(omega*RM)
 muzB = (-uM*sin(isMR) + wM*cos(isMR) )/(omega*RM) - viU/(omega*RM);    % m/s /(omega*RM)
  
 muyB = -muyB; % 左旋翼（顺时针）中的muyB作用与右旋翼（逆时针）相反
 
 % 3.体轴系桨毂处的角速度 转换到 桨毂轴系角速度（无量纲） 确定旋翼锥度角、后倒角和侧倾角,还有后向力系数与侧向力系数
 wxB  = ( p*cos(isMR) + r*sin(isMR) )/(omega);    % rad/s /(omega)
 wyB  = ( q )/(omega);
 %wzB  = (-pB*sin(isMR) + rB*cos(isMR) )/(omega);
 
 wxB  = -wxB; % 左旋翼（顺时针）中的wxB作用与右旋翼（逆时针）相反
 %wzB  = -wzB; % 转换为左旋翼坐标，wzB的方向相反
 
 % 4.初始化：确定UcB(垂直向下)，UtB(平行)
 CTB1 = 1; % CTB牛顿迭代初始值
 
 UcB  = -muzB / ( sqrt(kt*CTB1/2.d0) ); % sqrt(CT/2)*omega*R为悬停时候的诱导速度，UcB为风的速度，方向和桨毂运动速度相反，所以加上负号，搞不清楚可以假设前上飞，此时UcB一定大于0
 UtB  = sqrt(muxB^2 + muyB^2) / ( sqrt(kt*CTB1/2.d0) ); % 照道理也要添加负号，不过后面用的是Ut的平方，所以加不加负号无所谓
 
 % 5.初始化：确定诱导速度比
 if( (2.d0*UcB+3.d0)^2 + UtB*UtB >1.d0 )         % 滑流理论适用，Newton－Raphson方法迭代求解，Johson提出的涡环状态下经验估计
     viB = N_R ( UcB, UtB );                     % N_R为迭代函数
 else
     viB = UcB * ( 0.373d0*UcB*UcB + 0.598d0*UtB*UtB - 1.991d0 );
 end
 
 % 6.初始化：确定fG、lammda1(无量纲)、诱导速度和AEOCTB（代数方程右端项）
 %lammda = ( UcB+viB ) * sqrt(kt*CTB1/2.d0);                % 入流速度 /(omega*RM)
 %zh      = hB*k3*RM + HR - drotor;
 mu     = sqrt(muxB^2+muyB^2);                             % /(omega*RM)
 fG     = 1.0d0; %- sigmaMR*aMR*lammda/(4.d0*kt*CTB1) * (RM/(4.d0*z))**2/( 1.d0 + (mu/lammda)**2 )
 lammda1= muzB - viB * sqrt(kt*CTB1/2.d0) * fG * KindMR;  % 向下为正，若直升机向上飞 则muzB为负
  
 AEOCTB1  = kt*CTB1 - 0.5d0*kBLADE*aMR*sigmaMR*((1.d0/3.d0 + 0.5d0*mu^2)*theta0...
     + 0.25d0*(1.0d0 + mu^2)*theta1MR + 0.5d0*lammda1...
     - 0.5d0*(muyB*thetac + muxB*thetas) + 0.25d0*(muxB*wxB + muyB*wyB));  %  (与beta0, betac, betas无关，只与theta0, thetac, thetas有关)
 
 % 7.初始化：CTB2 = CTB1 + deltaCTB
 CTB2 = CTB1 + 1e-4;
 
 % 8.进入牛顿迭代：计算配平时候的CTB和vi
 for k = 1:10
     % 计算CTB2下的vi  
     UcB  = -muzB / ( sqrt(kt*CTB2/2.d0) );
     UtB  = sqrt(muxB^2 + muyB^2) / ( sqrt(kt*CTB2/2.d0) );
     if( (2.d0*UcB+3.d0)^2 + UtB*UtB >1.d0 )         
         viB = N_R ( UcB, UtB );                     
     else
         viB = UcB * ( 0.373d0*UcB*UcB + 0.598d0*UtB*UtB - 1.991d0 );
     end
     
     % 计算CTB2下的fG、lammda1(无量纲)、诱导速度和AEOCTB（代数方程右端项）
     %lammda = ( UcB+viB ) * sqrt(kt*CTB2/2.d0);            % 入流速度 /(omega*RM)
     %zh      = hB*k3*RM + HR - drotor;
     fG     = 1.d0 ;%- sigmaMR*aMR*lammda/(4.d0*kt*CTB1) * (RM/(4.d0*z))**2/( 1.d0 + (mu/lammda)**2 )
     lammda1= muzB - viB * sqrt(kt*CTB2/2.d0) * fG * KindMR;  % 向下为正，若直升机向上飞 则muzB为负
     
     AEOCTB2  = kt*CTB2 - 0.5d0*kBLADE*aMR*sigmaMR*((1.d0/3.d0 + 0.5d0*mu^2)*theta0...
         + 0.25d0*(1.0d0 + mu^2)*theta1MR + 0.5d0*lammda1...
         - 0.5d0*(muyB*thetac + muxB*thetas) + 0.25d0*(muxB*wxB + muyB*wyB));  %  (与beta0, betac, betas无关，只与theta0, thetac, thetas有关)
     
     dAEOCTB  =   (AEOCTB2 - AEOCTB1)/(CTB2-CTB1);
     
     AEOCTB1 = AEOCTB2;
     CTB1 = CTB2;
     CTBN = CTB2 - AEOCTB2/dAEOCTB;
     err = abs(CTBN-CTB2);
     relerr = 2*err/(abs(CTBN)+1e-4);
     CTB2 = CTBN;
     
%      % 新CTB2下的vi与AEOCTB（即y）
%      UcB  = -muzB / ( sqrt(kt*CTB2/2.d0) ); % sqrt(CT/2)*omega*R为悬停时候的诱导速度，UcB为风的速度，方向和桨毂运动速度相反，所以加上负号，搞不清楚可以假设前上飞，此时UcB一定大于0
%      UtB  = sqrt(muxB^2 + muyB^2) / ( sqrt(kt*CTB2/2.d0) ); % 照道理也要添加负号，不过后面用的是Ut的平方，所以加不加负号无所谓
%      if( (2.d0*UcB+3.d0)^2 + UtB*UtB >1.d0 )          % 滑流理论适用，Newton－Raphson方法迭代求解，Johson提出的涡环状态下经验估计
%          viB = N_R ( UcB, UtB );                      % N_R为迭代函数
%      else
%          viB = UcB * ( 0.373d0*UcB*UcB + 0.598d0*UtB*UtB - 1.991d0 );
%      end
%      %lammda = ( UcB+viB ) * sqrt(kt*CTB2/2.d0);     % 入流速度 /(omega*RM)
%      %zh      = hB*k3*RM + HR - drotor;
%      fG     = 1.d0 ;%- sigmaMR*aMR*lammda/(4.d0*kt*CTB1) * (RM/(4.d0*z))**2/( 1.d0 + (mu/lammda)**2 )
%      lammda1= muzB - viB * sqrt(kt*CTB2/2.d0) * fG * KindMR;                      % 向下为正，若直升机向上飞 则muzB为负
%      y = kt*CTB2 - 0.5d0*kBLADE*aMR*sigmaMR*((1.d0/3.d0 + 0.5d0*mu^2)*theta0...
%          + 0.25d0*(1.0d0 + mu^2)*theta1MR + 0.5d0*lammda1...
%          - 0.5d0*(muyB*thetac + muxB*thetas) + 0.25d0*(muxB*wxB + muyB*wyB));
     %if (err<1e-5)||(relerr<1e-5)||(abs(y)<1e-6)
     if (err<1e-4)||(relerr<1e-4)
         break;
     end
 end
 
 CTB = CTB2;
 vim = viB * sqrt(kt*CTB/2.d0) * fG * KindMR;
 viL = vim*omega*RM;
 
 AEOCTB = AEOCTB2;
 
 % 9.确定旋翼锥度角、后倒角和侧倾角(用于确定旋翼的后向力和侧向力) 
 Ca1     = 1.d0 - 0.5d0 * mu^2;
 Cb1     = 1.d0 + 0.5d0 * mu^2;
 
 beta0   = 0.5d0*kBLADE*gamaMR * ( 0.25d0*(1+mu^2)*theta0 + (0.2d0+ 1.d0/6.d0 *mu^2)*theta1MR ...
            - 1.d0/3.d0 *muyB*thetac - 1.d0/3.d0 *muxB*thetas + 1.d0/3.d0*lammda1 ...
            + 1.d0/6.d0 *muxB*wxB + 1.d0/6.d0 *muyB*wyB ) - g*MbMR/(IbMR * (omega)^2);
 
 betac   = (8.d0/3.d0 *theta0 + 2.d0*theta1MR + 2.d0*lammda1)*muxB/Ca1 ...
            - 2.d0*muxB*muyB/Ca1 *thetac - (Ca1+2.d0*muxB*muxB)/Ca1 *thetas ...
            + 4.0/(3.d0*Cb1) *muyB*beta0 ...
            + (Cb1 - muyB^2 + 16.d0/(gamaMR*kBLADE)*muxB*muyB) *wxB/(Ca1*Cb1) ...
            + (muxB*muyB - 16.d0/(gamaMR*kBLADE)*(Cb1 - muyB^2)) *wyB/(Ca1*Cb1);
 
 betas   = -(8.d0/3.d0 *theta0 + 2.d0*theta1MR + 2.d0*lammda1)*muyB/Ca1 ...
             + 2.d0*muxB*muyB/Ca1 *thetas + (Ca1+2.d0*muyB*muyB)/Ca1 *thetac ...
             + 4.0/(3.d0*Cb1) *muxB*beta0 ...
            - (Ca1 + muyB^2 - 16.d0/(gamaMR*kBLADE)*muxB*muyB) *wyB/(Ca1*Cb1) ...
            - (muxB*muyB + 16.d0/(gamaMR*kBLADE)*(Ca1 + muyB^2)) *wxB/(Ca1*Cb1);
 
 % 10.确定后向力系数、侧向力系数、需用功率
 CT = CTB*kt;
 
 CH      = 0.25d0*cdMRL*sigmaMR*muxB...   % (与beta0, betac, betas, theta0, thetac, thetas均有关)
            + 0.5d0*kBLADE*aMR*sigmaMR*( ...
            (-0.75d0*muyB *beta0 + (1.0/3.d0 + 0.5d0*muyB^2) *betac + 0.5d0*muxB*muyB *betas -0.5d0*muxB*lammda1 -1.d0/6.d0*wxB) *theta0 ...
            + 0.25d0*(-2.d0*muyB *beta0 + (1.d0+muyB^2) *betac + muxB*muyB *betas -muxB*lammda1 - 0.5d0*wxB) *theta1MR ...
            + 0.5d0*((1.d0/3.d0 + muyB^2)*beta0 - muyB*betac + 0.125d0*(muyB*wxB+muxB*wyB)) *thetac ...
            + 0.25d0*(2.d0*muxB*muyB*beta0 - muxB*betac - muyB*betas + lammda1 + 0.75d0*muxB*wxB + 0.25d0*muyB*wyB) *thetas ...
            - muxB*muyB*beta0*betac - (1.d0/6.d0-muyB*muyB)*beta0*betas - 0.25d0*muyB*betac*betas + 0.25d0*muxB*(beta0^2+betac^2) ...
            + 0.75d0*(betac-2.d0*muyB*beta0)*lammda1 ...
            - 0.5d0*(lammda1+0.125d0*muxB*betac-0.875d0*muyB*betas) *wxB - 0.5d0*(1.d0/3.d0*beta0-0.625d0*muyB*betac+0.125d0*muxB*betas) *wyB );
 
 CS      = -0.25d0*cdMRL*sigmaMR*muyB ... % (与beta0, betac, betas, theta0, thetac, thetas均有关)
            + 0.5d0*kBLADE*aMR*sigmaMR*( ...
            (-0.75d0*muxB *beta0 + (1.0/3.d0 + 0.5d0*muxB^2) *betas + 0.5d0*muxB*muyB *betac +0.5d0*muyB*lammda1 +1.d0/6.d0*wyB) *theta0 ...
            + 0.25d0*(-2.d0*muxB *beta0 + (1.d0+muxB^2) *betas + muxB*muyB *betac +muyB*lammda1 + 0.5d0*wyB) *theta1MR ...
            + 0.25d0*(2.d0*muxB*muyB *beta0 - muyB *betas - muxB *betac - lammda1 - 0.25d0*muxB*wxB - 0.75d0*muyB*wyB) *thetac ...
            + 0.5d0*((1.0/3.0 + muxB^2) *beta0 - muxB*betas -0.125d0*(muyB*wxB+muxB*wyB)) *thetas ...
            + muxB*muyB*beta0*betas + (1.d0/6.d0-muxB*muxB)*beta0*betac + 0.25d0*muxB*betac*betas - 0.25d0*muyB*(beta0^2+betas^2) ...
            + 0.75d0*(betas-2.d0*muxB*beta0)*lammda1 ...
            + 0.5d0*(lammda1-0.125d0*muyB*betas+0.875d0*muxB*betac) *wyB - 0.5d0*(1.d0/3.d0*beta0-0.625d0*muxB*betas+0.125d0*muyB*betac) *wxB );
 
 CHB      =  CH / kt;
 CSB      =  CS / kt;
  
 CpmB = (-CTB*muzB - CHB*muxB + CSB*muyB)/sqrt(kt) + KindMR*fG*CTB*sqrt(CTB/2.d0)*viB ...
         + 0.125d0*sigmaMR*cdMRL/kt/sqrt(kt)*(1.d0 + 4.7d0*mu^2);

 Cpm = CpmB*(kt*sqrt(kt));
      
 PSR = 1/eta*rho*(pi*RM^2)*(omega*RM)^3*Cpm;
 
 MMk = -PSR/omega;
 
 betas = -betas ; % 转换为右旋翼坐标，侧倒角betas的方向相反
 CS   = -CS;      % 转换为右旋翼坐标，侧向力系数CS的方向相反
  
 TLHK = nbMR/2.d0 * (XKBR)*betas;
 TMHK = nbMR/2.d0 * (XKBR)*betac;
 
 % 11.确定体轴系下的力和力矩
 FMx =  rho*(pi*RM^2)*(omega*RM)^2 * ( CT*sin(isMR) - CH*cos(isMR) );
 
 FMy =  rho*(pi*RM^2)*(omega*RM)^2 * CS;
 
 FMz = -rho*(pi*RM^2)*(omega*RM)^2 * ( CT*cos(isMR) + CH*sin(isMR) );
 
 MMx = 0.5*nbMR * MbMR * omega^2 * eMR * betas*cos(isMR) - MMk*sin(isMR)  + ( ym*FMz - zm*FMy ) + TLHK*cos(isMR);
 
 MMy = 0.5*nbMR * MbMR * omega^2 * eMR * betac + ( zm*FMx - xm*FMz ) + TMHK;
 
 MMz = 0.5*nbMR * MbMR * omega^2 * eMR * betas*sin(isMR) + MMk*cos(isMR)  + ( xm*FMy - ym*FMx ) + TLHK*sin(isMR);
 
 % 求诱导速度用到的函数
     function p0 = N_R(x_1B,x_2B)
         p0   = 1;
         delta= 0.0001;
         epsilon = 0.0001;
         max1 = 10;
         for k = 1:max1
             p1     = p0-( p0^4+2*x_1B*p0^3+(x_1B^2+x_2B^2)*p0^2-1 )/( 4*p0^3+6*x_1B*p0^2+2*(x_1B^2+x_2B^2)*p0 );
             err    = abs(p1-p0);
             relerr = 2*err/(abs(p1)+delta);
             p0     = p1;
             y      = p0^4+2*x_1B*p0^3+(x_1B^2+x_2B^2)*p0^2-1;
             if (err<delta)||(relerr<delta)||(abs(y)<epsilon)
                 break;
             end
         end

== matlab function eVTOL_Small_nonandlin_algorithm_validation/Subsystem1/MATLAB Function1 ==
  data: P output; t input
function P = faultRate(t)

if t < 220
    P = eye(16);
else
    % P = eye(16);

    V = [0.6, 1, 1, 1, 1, 1, 1, 1, 1, 1, 1, 1, 1, 1, 1, 1,];
    P = diag(V);
end

== matlab function eVTOL_Small_nonandlin_algorithm_validation/各部件气动力和力矩/机身/机身 ==
  data: u0 input; v0 input; w0 input; uW input; vW input; wW input; p input; q input; r input; xf input; yf input; zf input; FFx output; FFy output; FFz output; MFx output; MFy output; MFz output; rho input
 function [FFx, FFy, FFz, MFx, MFy, MFz] = FUSELAGE(u0,v0,w0,uW,vW,wW,p,q,r,xf,yf,zf,rho) 
 
 % 单位转换
 ft2m = 0.3048e0; 
 r2d  = 57.29577951e0;
 
 % 1.机身气动中心气流速度
 u = u0 + uW;
 v = v0/2.2 + vW/2.2;
 w = w0 + wW;
 
 uf = u + (zf*q - yf*r);
 vf = v + (xf*r - zf*p);
 wf = w + (yf*p - xf*q);
 
 % 2.机身风洞实验的迎角、侧滑角和实际的迎角、侧滑角的计算
 if (abs(uf) < 1.0e-10)
     if (abs(wf) < 1.0e-10)
         alfw = 0.0e0;
     else
         alfw = sign(wf)*pi/2.e0;
     end
     alff = alfw;
 elseif (uf > 0.0e0)
     alfw = atan(wf/uf);
     alff = alfw;
 else
     alfw = -atan(wf/uf);
     alff = sign(wf)*pi - alfw;
 end
             
 if (abs(uf) < 1.0e-10 && abs(wf) < 1.0e-10)
     if (abs(vf) < 1.0e-10)
         betaf = 0.0e0;
     else
         betaf = sign(vf)*pi/2.e0;
     end
 else
     betaf = atan(vf/sqrt(uf*uf + wf*wf));
 end
 
 % 3.由风洞实验得到的力和力矩系数
 psiw = -betaf;          % 力和力矩拟合相关参数确定
 salff  = sin(alff);
 calff  = cos(alff);
 sbetaf = sin(betaf);
 cbetaf = cos(betaf);
 salfw  = sin(alfw);
 calfw  = cos(alfw);
 spsiw  = sin(psiw);
 cpsiw  = cos(psiw);
 s2alfw = 2.e0*salfw*calfw;
 s2psiw = 2.e0*spsiw*cpsiw;
 c2psiw = 1.e0 - 2.e0*spsiw*spsiw;
 s4psiw = 2.e0*s2psiw*c2psiw;
 c4psiw = 1.e0 - 2.e0*s2psiw*s2psiw;
 psiwdeg = abs(psiw*r2d);
 
 CDq = ft2m^2 * (90.0555e0*salfw*salfw - 41.5604e0*calfw + 2.94684e0*c4psiw ...
     - 103.141e0*c2psiw - 0.535350e-6*(psiw*r2d)^4 + 160.2049e0) / 1.5;
 
 CLq = ft2m^2 * (29.3616e0*salfw + 43.4680e0*s2alfw - 81.8924e0*salfw*salfw - 84.1469e0*calfw ...
     - 0.0821406e0*psiw*r2d + 3.00102e0*s4psiw + 0.0323477e0*(psiw*r2d)^2 + 85.3496e0) / 200.e0;
 
 CYq = ft2m^2 * (35.3999e0*spsiw + 71.8019e0*s2psiw - 8.04823e0*s4psiw ) / 3;
 
 CMq = ft2m^3 * (2.37925e0*alfw*r2d + 728.026e0*s2alfw + 426.760e0*salfw*salfw ...
     + 348.072e0*calfw - 510.581e0*cpsiw^3 + 56.111e0) / 200.e0;
 
 if (psiwdeg <= 10.0e0)
     CRq = 0.0e0;                     % 滚转力矩
 elseif (psiwdeg <= 25.0e0)
     CRq = ft2m^3 * (455.707e0*cpsiw^4 - 428.639e0)*psiw*r2d/psiwdeg / 200.e0;
 else
     CRq = ft2m^3 * (614.797e0*spsiw + (-47.7213e0*c4psiw - 290.504e0*cpsiw^3 ...
         + 735.507e0*cpsiw^4 - 669.266e0)*psiw*r2d/psiwdeg) / 200.e0; 
 end
 
 if (psiwdeg <= 20.0e0)
     CNq = ft2m^3 * (-278.133e0*s2psiw + 422.644e0*s4psiw) / 200.e0; % 偏航
 else
     CNq = ft2m^3 * (220.0e0*s2psiw + (671.0e0*cpsiw^4 - 429.0e0)*psiw*r2d/psiwdeg) / 200.e0;
 end
                     
 DVF = 0.5*rho*(uf*uf + vf*vf + wf*wf);
 
 % 4.机身力和力矩的计算
 FFx =  0; %DVF*(-(CDq*cbetaf + CYq*sbetaf)*calff + CLq*salff );
 
 %FFx =  FFx/8; %不加机身外罩
 
 FFy =  0; %DVF*( -CDq*sbetaf + CYq*cbetaf );
 FFz =  0; %-DVF*( (CDq*cbetaf + CYq*sbetaf)*salff + CLq*calff );
 
 MFx =  0; %DVF*((CRq*cbetaf - CMq*sbetaf)*calff - CNq*salff) + (yf*FFz - zf*FFy);
 MFy =  0; %DVF* (CRq*sbetaf + CMq*cbetaf) + (zf*FFx - xf*FFz);
 MFz =  0; %DVF*((CRq*cbetaf - CMq*sbetaf)*salff + CNq*calff) + (xf*FFy - yf*FFx);

== matlab function eVTOL_Small_nonandlin_algorithm_validation/ControlAllocation 电机执行器 ==
  data: dt input; motorset output; de input; da input; dr input; Mc input
function  motorset = ControlAllocation(dt,de,da,dr, Mc)

% 控制指令dtB,de,da,dr转换为各个旋翼对应的油门，再转换为对应转速
% Dt_EXN = 1.15;

motor = [dt;de;da;dr];

motorset = Mc * motor;
